simulink model "MPCTracking"  (R2023b)
settings: Solver=VariableStepAuto  StartTime=0.0  StopTime=32  RelTol=1e-3
libraries: Solver_SF x1
settings Model: Creator=Lee  LastModifiedBy=Lee

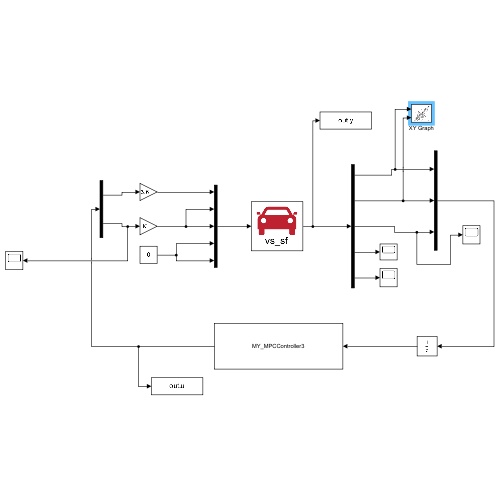
[thumbnail: Simulink's stored preview of the top-level diagram]
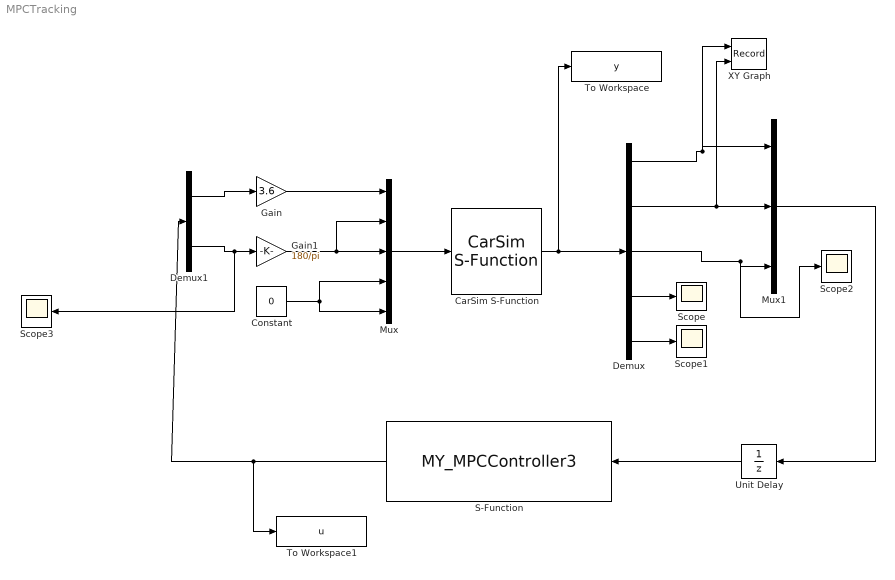
== system MPCTracking ==
  CarSim S-Function : Solver_SF/CarSim S-Function  Priority=1  SIMFILE=simfile.sim  Run_RTs=off  vs_state_ind=Run  StopMode_ind=Vehicle Model
  Constant : Constant  Value=0
  Demux : Demux  Outputs=5
  Demux1 : Demux  Outputs=2
  Gain : Gain  Gain=3.6
  Gain1 : Gain  Gain=180/pi
  Mux : Mux  Inputs=5
  Mux1 : Mux  Inputs=3
  S-Function : S-Function  FunctionName=MY_MPCController3  SFunctionDeploymentMode=off  EnableBusSupport=off
  Scope{,1..3} (4 alike) : Scope
  To Workspace : ToWorkspace  VariableName=y  SaveFormat=Structure  SampleTime=-1
  To Workspace1 : ToWorkspace  VariableName=u  SaveFormat=Structure  SampleTime=-1
  Unit Delay : UnitDelay  SampleTime=-1  HasFrameUpgradeWarning=on
  XY Graph : Record  FileSettingsInternal="{\"entries\":[{\"content\":{\"excelSettings\":{\"content\":{},\"type\":\"Streamout.ExcelSettings\"}},\"type\":\"Streamout.FileSettingStorage\",\"uuid\":\"\"}],\"packageUris\":[\"http:\\/\\/schema.mathworks.com\\/mf0\\/streamout_blocks\\/R2020a\"],\"version\":\"1.0\"}"  Layout=[1 1]  SignalsInternal="{\"entries\":[{\"content\":{\"signals\":[{\"content\":{\"blockPath\":[],\"dimensions\":[1],\"domain\":\"\",\"lineColor\":\"#a2142f\",\"plots\":[ 1 ],\"port\":1,\"sid\":[\"\"],\"signalID\":1,\"signalName\":\"Demux:1\"},\"type\":\"RecordBlkView.Signal\",\"uuid\":\"\"},{\"content\":{\"blockPath\":[],\"dimensions\":[1],\"domain\":\"\",\"lineColor\":\"#139fff\",\"plots\":[ 1 ],\"port\":2,\"sid\":[\"\"],\"signalID\":2,\"signalName\":\"Demux:2\"},\"type\":\"RecordBlkView.Signal\",\"uuid\":\"\"}]},\"type\":\"RecordBlkView.InputSignals\",\"uuid\":\"\"}],\"packageUris\":[\"http:\\/\\/schema.mathworks.com\\/mf0\\/streamout_blocks\\/R2020a\"],\"version\":\"1.0\"}"  VisualizationBindings="{\"xyplotplugin\":{\"info\":[{\"series\":[{\"bindingParametersList\":[{\"parameter\":\"X-Axis\",\"signalID\":1,\"signalName\":\"Demux:1\"},{\"parameter\":\"Y-Axis\",\"signalID\":2,\"signalName\":\"Demux:2\"}],\"seriesID\":0}],\"subplotID\":1}]}}"  CompatibilityTag=XY
  wires:
  CarSim S-Function/1 -> To Workspace/1, Demux/1
  Mux/1 -> CarSim S-Function/1
  Gain/1 -> Mux/1
  Gain1/1 -> Mux/2, Mux/3
  Constant/1 -> Mux/5, Mux/4
  Demux1/1 -> Gain/1
  Demux1/2 -> Scope3/1, Gain1/1
  S-Function/1 -> To Workspace1/1, Demux1/1
  Demux/2 -> Mux1/2, XY Graph/2
  Demux/1 -> XY Graph/1, Mux1/1
  Demux/3 -> Scope2/1, Mux1/3
  Unit Delay/1 -> S-Function/1
  Mux1/1 -> Unit Delay/1
  Demux/4 -> Scope/1
  Demux/5 -> Scope1/1
